simulink model "FSFB_model"  (R2016b)
settings: Solver=ode45  StartTime=0.0  StopTime=t_final  RelTol=1e-3  EnableMultiTasking=on
values from neighbouring files (symbols this model uses):
  A = [0 1 0 ... (first row only)    [lecture_PracticalFSFB.m]    (also in lecture_eigenvalue_for_FSFB.m)
  Acl = A-B1*K    [lecture_PracticalFSFB.m]
  B = [0 0 ... (first row only)    [lecture_PracticalFSFB.m]    (also in lecture_eigenvalue_for_FSFB.m)
  C = eye(3)    [lecture_PracticalFSFB.m]
  D = zeros(3,2)    [lecture_PracticalFSFB.m]
  K = place(A,B1,desired_closed_loop_poles)    [lecture_PracticalFSFB.m]
  x0 = [72*pi/180 ... (first row only)    [lecture_PracticalFSFB.m]
settings Model: Creator=lum  LastModifiedBy=Christopher
settings DataIOCC: LimitDataPoints=on  SaveFormat=Array  SignalLoggingSaveFormat=ModelDataLogs
settings OptimizationCC: ExpressionDepthLimit=2147483647  InitFltsAndDblsToZero=on  LifeSpan=inf
settings DebuggingCC: SaveWithParameterizedLinksMsg=none  UnderspecifiedInitializationDetection=Classic  MergeDetectMultiDrivingBlocksExec=none  SolverPrmCheckMsg=warning  FcnCallInpInsideContextMsg=warning  StateNameClashWarn=warning  SFUnexpectedBacktrackingDiag=warning  SFNoUnconditionalDefaultTransitionDiag=warning  SFExecutionAtInitializationDiag=none
settings HardwareCC: ProdBitPerPointer=32  ProdBitPerSizeT=32  ProdBitPerPtrDiffT=32  ProdLargestAtomicFloat=None  ProdIntDivRoundTo=Undefined  ProdEndianess=Unspecified  ProdWordSize=32  ProdHWDeviceType=32-bit Generic
settings ModelReferenceCC: PropagateSignalLabelsOutOfModel=off
settings GRTTargetCC: TargetFcnLib=ansi_tfl_tmw.mat  TargetLangStandard=C89/C90 (ANSI)  GeneratePreprocessorConditionals=Disable all  CombineOutputUpdateFcns=off  GRTInterface=on
settings ConfigComp: CovMetricSettings=dw  CovHtmlReporting=on  CovSaveCumulativeToWorkspaceVar=on  CovSaveSingleToWorkspaceVar=on  CovExternalEMLEnable=off

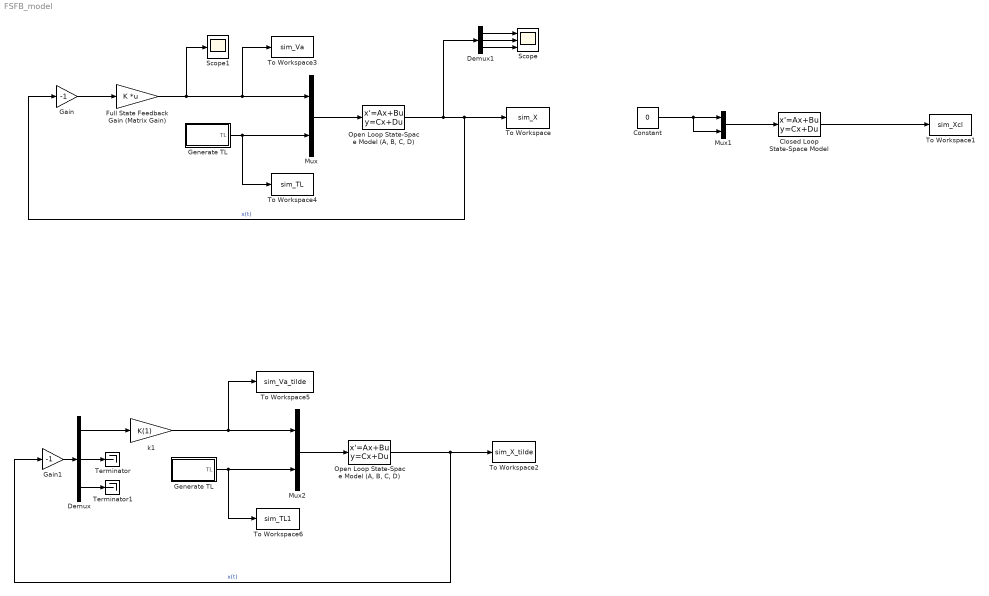
== system FSFB_model ==
  Closed Loop State-Space Model : StateSpace  A=Acl  B=zeros(3,2)  C=eye(3)  D=zeros(3,2)  X0=x0
  Constant : Constant  Value=0
  Demux : Demux  Outputs=3
  Demux1 : Demux  Outputs=3
  Full State Feedback Gain (Matrix Gain) : Gain  Gain=K  Multiplication=Matrix(K*u)
  Gain : Gain  Gain=-1
  Gain1 : Gain  Gain=-1
  Generate TL : Subsystem
  "Generate TL " : Subsystem
  Mux : Mux  Inputs=2
  Mux1 : Mux  Inputs=2
  Mux2 : Mux  Inputs=2
  "Open Loop State-Space Model (A, B, C, D)" : StateSpace  A=A  B=B  C=C  D=D  X0=x0
  "Open Loop State-Space Model (A, B, C, D) " : StateSpace  A=A  B=B  C=C  D=D  X0=x0
  Scope : Scope  NumInputPorts=3
  Scope1 : Scope
  Terminator : Terminator
  Terminator1 : Terminator
  To Workspace : ToWorkspace  VariableName=sim_X  SaveFormat=Structure With Time  SampleTime=-1
  To Workspace1 : ToWorkspace  VariableName=sim_Xcl  SaveFormat=Structure With Time  SampleTime=-1
  To Workspace2 : ToWorkspace  VariableName=sim_X_tilde  SaveFormat=Structure With Time  SampleTime=-1
  To Workspace3 : ToWorkspace  VariableName=sim_Va  SaveFormat=Structure With Time  SampleTime=-1
  To Workspace4 : ToWorkspace  VariableName=sim_TL  SaveFormat=Structure With Time  SampleTime=-1
  To Workspace5 : ToWorkspace  VariableName=sim_Va_tilde  SaveFormat=Structure With Time  SampleTime=-1
  To Workspace6 : ToWorkspace  VariableName=sim_TL1  SaveFormat=Structure With Time  SampleTime=-1
  k1 : Gain  Gain=K(1)
  wires:
  Full State Feedback Gain (Matrix Gain)/1 -> To Workspace3/1, Mux/1, Scope1/1
  "Open Loop State-Space Model (A, B, C, D)"/1 -> To Workspace/1, Gain/1, Demux1/1  "x(t)"
  Generate TL/1(TL) -> To Workspace4/1, Mux/2
  Gain/1 -> Full State Feedback Gain (Matrix Gain)/1
  Mux/1 -> "Open Loop State-Space Model (A, B, C, D)"/1
  Closed Loop State-Space Model/1 -> To Workspace1/1
  Mux1/1 -> Closed Loop State-Space Model/1
  Constant/1 -> Mux1/1, Mux1/2
  k1/1 -> Mux2/1, To Workspace5/1
  "Open Loop State-Space Model (A, B, C, D) "/1 -> Gain1/1, To Workspace2/1  "x(t)"
  "Generate TL "/1(TL) -> Mux2/2, To Workspace6/1
  Gain1/1 -> Demux/1
  Mux2/1 -> "Open Loop State-Space Model (A, B, C, D) "/1
  Demux/1 -> k1/1
  Demux/2 -> Terminator/1
  Demux/3 -> Terminator1/1
  Demux1/1 -> Scope/1
  Demux1/2 -> Scope/2
  Demux1/3 -> Scope/3

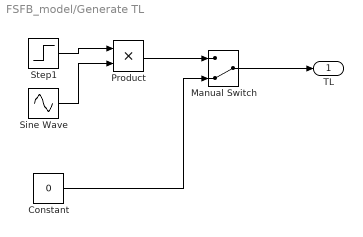
== system FSFB_model/Generate TL ==
  Constant : Constant  Value=0
  Manual Switch : ManualSwitch  CurrentSetting=0
  Product : Product  RndMeth=Zero
  Sine Wave : Sin  SampleTime=0
  Step1 : Step  Time=3  SampleTime=0
  TL : Outport
  wires:
  Step1/1 -> Product/1
  Sine Wave/1 -> Product/2
  Product/1 -> Manual Switch/1
  Manual Switch/1 -> TL/1
  Constant/1 -> Manual Switch/2

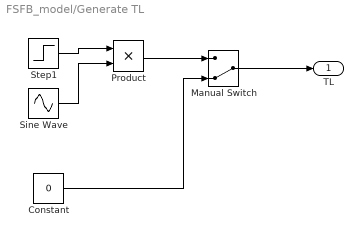
== system FSFB_model/Generate TL  ==
  Constant : Constant  Value=0
  Manual Switch : ManualSwitch  CurrentSetting=0
  Product : Product  RndMeth=Zero
  Sine Wave : Sin  SampleTime=0
  Step1 : Step  Time=3  SampleTime=0
  TL : Outport
  wires:
  Constant/1 -> Manual Switch/2
  Manual Switch/1 -> TL/1
  Product/1 -> Manual Switch/1
  Sine Wave/1 -> Product/2
  Step1/1 -> Product/1
